simulink model "singlcontact_control_smc_lqr_mydimes_reaction"  (R2024a)
settings: Solver=VariableStepAuto  StartTime=0.0  StopTime=10  FixedStep=0.001  RelTol=1e-3
values from neighbouring files (symbols this model uses):
  ankle_servo_kd = 8    [robotParametersCtrl_mydiem_block_zmp.m]    (also in robotParametersCtrl_quad_modify_mydiem.m; robotParametersCtrl_quad_modify_mydiem_reaction.m)
  ankle_servo_ki = 4    [robotParametersCtrl_mydiem_block_zmp.m]    (also in robotParametersCtrl_quad_modify_mydiem.m; robotParametersCtrl_quad_modify_mydiem_reaction.m)
  ankle_servo_kp = 20    [robotParametersCtrl_mydiem_block_zmp.m]    (also in robotParametersCtrl_quad_modify_mydiem.m; robotParametersCtrl_quad_modify_mydiem_reaction.m)
  deriv_filter_coeff = 100    [robotParametersCtrl_mydiem_block_zmp.m]    (also in robotParametersCtrl_quad_modify_mydiem.m; robotParametersCtrl_quad_modify_mydiem_reaction.m)
  filter_coefficent_pid = 100    [robotParametersCtrl_mydiem_block_zmp.m]    (also in robotParametersCtrl_quad_modify_mydiem.m; robotParametersCtrl_quad_modify_mydiem_reaction.m)
  filter_coefficent_pids = 100    [robotParametersCtrl_quad_modify_mydiem_reaction.m]
  foot_z = 1.5    [robotParametersCtrl_mydiem_block_zmp.m]    (also in robotParametersCtrl_quad_modify_mydiem.m; robotParametersCtrl_quad_modify_mydiem_reaction.m)
  g = 9.81    [ABCDvalues_lqr_quad_mydime_reaction.m]    (also in robotParametersCtrl_mydiem_block_zmp.m = 9.80665; robotParametersCtrl_quad_modify_mydiem.m = 9.80665; robotParametersCtrl_quad_modify_mydiem_reaction.m = 9.80665)
  h = 32    [robotParametersCtrl_mydiem_block_zmp.m]    (also in robotParametersCtrl_quad_modify_mydiem.m; robotParametersCtrl_quad_modify_mydiem_reaction.m)
  height_plane = 0.025    [robotParametersCtrl_mydiem_block_zmp.m]    (also in robotParametersCtrl_quad_modify_mydiem.m; robotParametersCtrl_quad_modify_mydiem_reaction.m)
  hip_pitch_deriv = 20    [robotParametersCtrl_mydiem_block_zmp.m]    (also in robotParametersCtrl_quad_modify_mydiem.m = 200; robotParametersCtrl_quad_modify_mydiem_reaction.m = 200)
  hip_pitch_derivs = 200    [robotParametersCtrl_quad_modify_mydiem_reaction.m]
  hip_pitch_int = 0    [robotParametersCtrl_mydiem_block_zmp.m]    (also in robotParametersCtrl_quad_modify_mydiem.m = 150; robotParametersCtrl_quad_modify_mydiem_reaction.m = 150)
  hip_pitch_ints = 1500    [robotParametersCtrl_quad_modify_mydiem_reaction.m]
  hip_pitch_prop = 10    [robotParametersCtrl_mydiem_block_zmp.m]    (also in robotParametersCtrl_quad_modify_mydiem.m = 500; robotParametersCtrl_quad_modify_mydiem_reaction.m = 500)
  hip_pitch_props = 500    [robotParametersCtrl_quad_modify_mydiem_reaction.m]
  hip_roll_deriv = 28    [robotParametersCtrl_mydiem_block_zmp.m]    (also in robotParametersCtrl_quad_modify_mydiem.m = 280; robotParametersCtrl_quad_modify_mydiem_reaction.m = 280)
  hip_roll_derivs = 280    [robotParametersCtrl_quad_modify_mydiem_reaction.m]
  hip_roll_int = 0    [robotParametersCtrl_mydiem_block_zmp.m]    (also in robotParametersCtrl_quad_modify_mydiem.m = 180; robotParametersCtrl_quad_modify_mydiem_reaction.m = 180)
  hip_roll_ints = 180    [robotParametersCtrl_quad_modify_mydiem_reaction.m]
  hip_roll_prop = 10    [robotParametersCtrl_mydiem_block_zmp.m]    (also in robotParametersCtrl_quad_modify_mydiem.m = 300; robotParametersCtrl_quad_modify_mydiem_reaction.m = 300)
  hip_roll_props = 300    [robotParametersCtrl_quad_modify_mydiem_reaction.m]
  hip_servo_kd = 20    [robotParametersCtrl_mydiem_block_zmp.m]    (also in robotParametersCtrl_quad_modify_mydiem.m; robotParametersCtrl_quad_modify_mydiem_reaction.m)
  hip_servo_ki = 10    [robotParametersCtrl_mydiem_block_zmp.m]    (also in robotParametersCtrl_quad_modify_mydiem.m; robotParametersCtrl_quad_modify_mydiem_reaction.m)
  hip_servo_kp = 60    [robotParametersCtrl_mydiem_block_zmp.m]    (also in robotParametersCtrl_quad_modify_mydiem.m; robotParametersCtrl_quad_modify_mydiem_reaction.m)
  hip_smc_lamda = 85    [robotParametersCtrl_mydiem_block_zmp.m]    (also in robotParametersCtrl_quad_modify_mydiem.m; robotParametersCtrl_quad_modify_mydiem_reaction.m = 95)
  hip_smc_lamdas = 85    [robotParametersCtrl_quad_modify_mydiem_reaction.m]
  hip_smc_new = 25    [robotParametersCtrl_mydiem_block_zmp.m]    (also in robotParametersCtrl_quad_modify_mydiem.m; robotParametersCtrl_quad_modify_mydiem_reaction.m = 45)
  hip_smc_news = 25    [robotParametersCtrl_quad_modify_mydiem_reaction.m]
  init_angs_L = init_angs_R    [robotParametersCtrl_mydiem_block_zmp.m]    (also in robotParametersCtrl_quad_modify_mydiem.m; robotParametersCtrl_quad_modify_mydiem_reaction.m)
  init_angs_R = [0 -sum(init_angs) init_angs(2) 0 init_angs(1)]    [robotParametersCtrl_mydiem_block_zmp.m]    (also in robotParametersCtrl_quad_modify_mydiem.m; robotParametersCtrl_quad_modify_mydiem_reaction.m)
  init_height = h +                torso_z/2 + torso_offset_z + height_plane/2    (= 39.5125)    [robotParametersCtrl_mydiem_block_zmp.m]    (also in robotParametersCtrl_quad_modify_mydiem.m; robotParametersCtrl_quad_modify_mydiem_reaction.m)
  K = lqr(A, B, Q, R)    [ABCDvalues_lqr_quad_mydime_reaction.m]
  knee_pitch_deriv = 10    [robotParametersCtrl_mydiem_block_zmp.m]    (also in robotParametersCtrl_quad_modify_mydiem.m = 100; robotParametersCtrl_quad_modify_mydiem_reaction.m = 100)
  knee_pitch_derivs = 180    [robotParametersCtrl_quad_modify_mydiem_reaction.m]
  knee_pitch_int = 0    [robotParametersCtrl_mydiem_block_zmp.m]    (also in robotParametersCtrl_quad_modify_mydiem.m = 300; robotParametersCtrl_quad_modify_mydiem_reaction.m = 300)
  knee_pitch_ints = 7500    [robotParametersCtrl_quad_modify_mydiem_reaction.m]
  knee_pitch_prop = 10    [robotParametersCtrl_mydiem_block_zmp.m]    (also in robotParametersCtrl_quad_modify_mydiem.m = 400; robotParametersCtrl_quad_modify_mydiem_reaction.m = 400)
  knee_pitch_props = 1200    [robotParametersCtrl_quad_modify_mydiem_reaction.m]
  knee_servo_kd = 10    [robotParametersCtrl_mydiem_block_zmp.m]    (also in robotParametersCtrl_quad_modify_mydiem.m; robotParametersCtrl_quad_modify_mydiem_reaction.m)
  knee_servo_ki = 5    [robotParametersCtrl_mydiem_block_zmp.m]    (also in robotParametersCtrl_quad_modify_mydiem.m; robotParametersCtrl_quad_modify_mydiem_reaction.m)
  knee_servo_kp = 60    [robotParametersCtrl_mydiem_block_zmp.m]    (also in robotParametersCtrl_quad_modify_mydiem.m; robotParametersCtrl_quad_modify_mydiem_reaction.m)
  knee_smc_lamda = 140    [robotParametersCtrl_mydiem_block_zmp.m]    (also in robotParametersCtrl_quad_modify_mydiem.m; robotParametersCtrl_quad_modify_mydiem_reaction.m = 150)
  knee_smc_lamdas = 100    [robotParametersCtrl_quad_modify_mydiem_reaction.m]
  knee_smc_new = 80    [robotParametersCtrl_mydiem_block_zmp.m]    (also in robotParametersCtrl_quad_modify_mydiem.m; robotParametersCtrl_quad_modify_mydiem_reaction.m)
  knee_smc_news = 60    [robotParametersCtrl_quad_modify_mydiem_reaction.m]
  Kwalk = 0.6    [robotParametersCtrl_mydiem_block_zmp.m]    (also in robotParametersCtrl_quad_modify_mydiem.m; robotParametersCtrl_quad_modify_mydiem_reaction.m)
  l1 = 0.20    (= 0.2)    [ABCDvalues_lqr_quad_mydime_reaction.m]
  l2 = 0.20    (= 0.2)    [ABCDvalues_lqr_quad_mydime_reaction.m]
  lower_leg_length = 20    [robotParametersCtrl_mydiem_block_zmp.m]    (also in robotParametersCtrl_quad_modify_mydiem.m; robotParametersCtrl_quad_modify_mydiem_reaction.m)
  m1 = 0.45    [ABCDvalues_lqr_quad_mydime_reaction.m]
  m2 = 0.065    [ABCDvalues_lqr_quad_mydime_reaction.m]
  max_torque = 20    [robotParametersCtrl_mydiem_block_zmp.m]    (also in robotParametersCtrl_quad_modify_mydiem.m; robotParametersCtrl_quad_modify_mydiem_reaction.m)
  motion_time_constant = 0.01    [robotParametersCtrl_mydiem_block_zmp.m]    (also in robotParametersCtrl_quad_modify_mydiem.m; robotParametersCtrl_quad_modify_mydiem_reaction.m)
  plane_x = 25    [robotParametersCtrl_mydiem_block_zmp.m]    (also in robotParametersCtrl_quad_modify_mydiem.m; robotParametersCtrl_quad_modify_mydiem_reaction.m)
  plane_y = 3    [robotParametersCtrl_mydiem_block_zmp.m]    (also in robotParametersCtrl_quad_modify_mydiem.m; robotParametersCtrl_quad_modify_mydiem_reaction.m)
  stepHeight = 0.4    [ABCDvalues_lqr_quad_mydime_reaction.m]
  torso_offset_x = 17    [robotParametersCtrl_mydiem_block_zmp.m]    (also in robotParametersCtrl_quad_modify_mydiem.m; robotParametersCtrl_quad_modify_mydiem_reaction.m)
  torso_offset_x1 = -17    [robotParametersCtrl_mydiem_block_zmp.m]    (also in robotParametersCtrl_quad_modify_mydiem.m; robotParametersCtrl_quad_modify_mydiem_reaction.m)
  torso_offset_z = 0    [robotParametersCtrl_mydiem_block_zmp.m]    (also in robotParametersCtrl_quad_modify_mydiem.m; robotParametersCtrl_quad_modify_mydiem_reaction.m)
  torso_x = 40    [robotParametersCtrl_mydiem_block_zmp.m]    (also in robotParametersCtrl_quad_modify_mydiem.m; robotParametersCtrl_quad_modify_mydiem_reaction.m)
  torso_y = 20    [robotParametersCtrl_mydiem_block_zmp.m]    (also in robotParametersCtrl_quad_modify_mydiem.m; robotParametersCtrl_quad_modify_mydiem_reaction.m)
  torso_z = 15    [robotParametersCtrl_mydiem_block_zmp.m]    (also in robotParametersCtrl_quad_modify_mydiem.m; robotParametersCtrl_quad_modify_mydiem_reaction.m)
  Ts = 0.05    [ABCDvalues_lqr_quad_mydime_reaction.m]
  TsCtrl = 0.05    [robotParametersCtrl_mydiem_block_zmp.m]    (also in robotParametersCtrl_quad_modify_mydiem.m; robotParametersCtrl_quad_modify_mydiem_reaction.m)
  tWalk = 0.3    [robotParametersCtrl_mydiem_block_zmp.m]    (also in robotParametersCtrl_quad_modify_mydiem.m; robotParametersCtrl_quad_modify_mydiem_reaction.m)
  upper_leg_length = 20    [robotParametersCtrl_mydiem_block_zmp.m]    (also in robotParametersCtrl_quad_modify_mydiem.m; robotParametersCtrl_quad_modify_mydiem_reaction.m)
undefined symbols (not defined in the file or in its folder): X, Y, Z
libraries: simulink_extras x256, slpidlib x128, sm_lib x71, simulink x43, nesl_utility x35, walkingRobotUtils x21, dspsrcs4 x18, dspobslib x8
(part 31 of 33)

== system singlcontact_control_smc_lqr_mydimes_reaction/Walking Robot/smc+neuro+distur1/SMC Controllers FR2/Equivalent control/SMC equivalent T1 ==
  theta2 : Inport
  theta1 : Inport  Port=2
  theta2ddot : Inport  Port=3
  theta1dot : Inport  Port=4
  theta2dot : Inport  Port=5
  theta1ddot : Inport  Port=6
  Add{1..4} (4 alike) : Sum
  Add5 : Sum  Inputs=+--+++
  Add6 : Sum  Inputs=++++
  Constant : Constant  Value=0.3
  Constant10 : Constant  Value=m2*l1^2
  Constant11 : Constant  Value=0.3*m1*l1^2
  Constant12 : Constant  Value=m2*l1*l2
  Constant2 : Constant  Value=0.5
  Constant3 : Constant
  Constant4 : Constant  Value=0.5
  Constant5 : Constant
  Constant6 : Constant  Value=g*l1
  Constant7 : Constant  Value=0.5
  Constant9 : Constant  Value=0.3*m2*l2^2
  Cos : Trigonometry  Operator=cos
  Cos1 : Trigonometry  Operator=cos
  Gain1 : Gain  Gain=m2*l2^2
  Gain2 : Gain  Gain=m2*l2*l1
  Gain4 : Gain  Gain=m2*l2*l1
  Gain6 : Gain  Gain=m1
  Gain7 : Gain  Gain=m2
  Gain8 : Gain  Gain=m2*g*l2
  Product{1..3,7..9} (6 alike) : Product
  Product4 : Product  Inputs=4
  Product5 : Product  Inputs=3
  Product6 : Product  Inputs=3
  Sin : Trigonometry
  Sin1 : Trigonometry
  Sin2 : Trigonometry
  Square1 : Math  Operator=square
  T1 : Outport
  wires:
  Add2/1 -> Product1/1
  Product9/1 -> Add2/2
  [lamdaBR1] -> Product9/1
  [edotBR1] -> Product9/2
  Add5/1 -> T1/1
  Product1/1 -> Add5/6
  theta1ddot/1 -> Add2/1
  Add6/1 -> Product1/2
  Product8/1 -> Add6/1
  Constant11/1 -> Add6/2
  Constant10/1 -> Add6/4
  Constant9/1 -> Add6/3
  Cos1/1 -> Product8/1
  Constant12/1 -> Product8/2  "X_dd"
  theta2/1 -> Cos/1, Sin/1, Add4/1, Cos1/1
  Product7/1 -> Add5/5
  Product6/1 -> Add5/4
  Product5/1 -> Add5/3
  Product4/1 -> Add5/2
  Product3/1 -> Add5/1
  Sin2/1 -> Product7/2
  Gain8/1 -> Product7/1
  Add4/1 -> Sin2/1
  Constant7/1 -> Gain8/1
  Constant6/1 -> Product6/3
  Sin1/1 -> Product6/2
  Add3/1 -> Product6/1
  theta1/1 -> Sin1/1, Add4/2
  Gain6/1 -> Add3/1
  Gain7/1 -> Add3/2
  Constant5/1 -> Gain7/1
  Constant4/1 -> Gain6/1
  Square1/1 -> Product5/3
  Constant3/1 -> Gain4/1
  Gain4/1 -> Product4/1
  Sin/1 -> Product5/2, Product4/2
  theta2dot/1 -> Square1/1, Product4/4
  theta1dot/1 -> Product4/3
  Add1/1 -> Product3/2
  theta2ddot/1 -> Product3/1
  Product2/1 -> Add1/2
  Gain1/1 -> Add1/1
  Gain2/1 -> Product5/1, Product2/1
  Cos/1 -> Product2/2
  Constant2/1 -> Gain2/1
  Constant/1 -> Gain1/1

== system singlcontact_control_smc_lqr_mydimes_reaction/Walking Robot/smc+neuro+distur1/SMC Controllers FR2/Equivalent control/SMC equivalent T2 ==
  theta1ddot : Inport
  theta2 : Inport  Port=2
  theta1 : Inport  Port=3
  theta2ddot : Inport  Port=4
  theta1dot : Inport  Port=5
  Add1 : Sum
  Add2 : Sum
  Add4 : Sum
  Add5 : Sum  Inputs=++++
  Constant : Constant  Value=0.5
  Constant1 : Constant  Value=0.3
  Constant2 : Constant  Value=0.5
  Constant3 : Constant
  Gain10 : Gain  Gain=m2*l2^2
  Gain11 : Gain  Gain=m2*l2
  Gain12 : Gain  Gain=g
  Gain13 : Gain  Gain=(1/3)*(m2*(l2^2))
  Gain5 : Gain  Gain=m2*l1*l2
  Product{1..4,7} (5 alike) : Product
  Product6 : Product  Inputs=3
  Sin : Trigonometry
  Square3 : Math  Operator=square
  Trigonometric Function3 : Trigonometry  Operator=cos
  Trigonometric Function4 : Trigonometry
  T2 : Outport
  wires:
  Product2/1 -> Add5/4
  Gain13/1 -> Product2/1
  Add1/1 -> Product2/2
  Constant3/1 -> Gain13/1
  theta2ddot/1 -> Add1/2
  [edotBR2] -> Product1/1
  [lamdaBR2] -> Product1/2
  Product1/1 -> Add1/1
  Add5/1 -> T2/1
  Product7/1 -> Add5/3
  Product6/1 -> Add5/2
  Product4/1 -> Add5/1
  Add4/1 -> Sin/1
  Sin/1 -> Product7/2
  theta1/1 -> Add4/1
  Gain12/1 -> Product7/1
  Gain11/1 -> Gain12/1
  Constant2/1 -> Gain11/1
  Square3/1 -> Product6/3
  theta1dot/1 -> Square3/1
  Trigonometric Function4/1 -> Product6/2
  Constant1/1 -> Gain10/1
  Constant/1 -> Gain5/1
  theta1ddot/1 -> Product4/1
  Add2/1 -> Product4/2
  Gain10/1 -> Add2/2
  Product3/1 -> Add2/1
  Gain5/1 -> Product6/1, Product3/2
  Trigonometric Function3/1 -> Product3/1
  theta2/1 -> Trigonometric Function4/1, Add4/2, Trigonometric Function3/1

== system singlcontact_control_smc_lqr_mydimes_reaction/Walking Robot/smc+neuro+distur1/SMC Controllers FR3/Equivalent control/SMC equivalent T1 ==
  theta2 : Inport
  theta1 : Inport  Port=2
  theta2ddot : Inport  Port=3
  theta1dot : Inport  Port=4
  theta2dot : Inport  Port=5
  theta1ddot : Inport  Port=6
  Add{1..4} (4 alike) : Sum
  Add5 : Sum  Inputs=+--+++
  Add6 : Sum  Inputs=++++
  Constant : Constant  Value=0.3
  Constant10 : Constant  Value=m2*l1^2
  Constant11 : Constant  Value=0.3*m1*l1^2
  Constant12 : Constant  Value=m2*l1*l2
  Constant2 : Constant  Value=0.5
  Constant3 : Constant
  Constant4 : Constant  Value=0.5
  Constant5 : Constant
  Constant6 : Constant  Value=g*l1
  Constant7 : Constant  Value=0.5
  Constant9 : Constant  Value=0.3*m2*l2^2
  Cos : Trigonometry  Operator=cos
  Cos1 : Trigonometry  Operator=cos
  Gain1 : Gain  Gain=m2*l2^2
  Gain2 : Gain  Gain=m2*l2*l1
  Gain4 : Gain  Gain=m2*l2*l1
  Gain6 : Gain  Gain=m1
  Gain7 : Gain  Gain=m2
  Gain8 : Gain  Gain=m2*g*l2
  Product{1..3,7..9} (6 alike) : Product
  Product4 : Product  Inputs=4
  Product5 : Product  Inputs=3
  Product6 : Product  Inputs=3
  Sin : Trigonometry
  Sin1 : Trigonometry
  Sin2 : Trigonometry
  Square1 : Math  Operator=square
  T1 : Outport
  wires:
  Constant/1 -> Gain1/1
  Constant2/1 -> Gain2/1
  Cos/1 -> Product2/2
  Gain2/1 -> Product2/1, Product5/1
  Gain1/1 -> Add1/1
  Product2/1 -> Add1/2
  theta2ddot/1 -> Product3/1
  Add1/1 -> Product3/2
  theta1dot/1 -> Product4/3
  theta2dot/1 -> Product4/4, Square1/1
  Sin/1 -> Product4/2, Product5/2
  Gain4/1 -> Product4/1
  Constant3/1 -> Gain4/1
  Square1/1 -> Product5/3
  Constant4/1 -> Gain6/1
  Constant5/1 -> Gain7/1
  Gain7/1 -> Add3/2
  Gain6/1 -> Add3/1
  theta1/1 -> Add4/2, Sin1/1
  Add3/1 -> Product6/1
  Sin1/1 -> Product6/2
  Constant6/1 -> Product6/3
  Constant7/1 -> Gain8/1
  Add4/1 -> Sin2/1
  Gain8/1 -> Product7/1
  Sin2/1 -> Product7/2
  Product3/1 -> Add5/1
  Product4/1 -> Add5/2
  Product5/1 -> Add5/3
  Product6/1 -> Add5/4
  Product7/1 -> Add5/5
  theta2/1 -> Cos1/1, Add4/1, Sin/1, Cos/1
  Constant12/1 -> Product8/2  "X_dd"
  Cos1/1 -> Product8/1
  Constant9/1 -> Add6/3
  Constant10/1 -> Add6/4
  Constant11/1 -> Add6/2
  Product8/1 -> Add6/1
  Add6/1 -> Product1/2
  theta1ddot/1 -> Add2/1
  Product1/1 -> Add5/6
  Add5/1 -> T1/1
  [edotBL1] -> Product9/2
  [lamdaBL1] -> Product9/1
  Product9/1 -> Add2/2
  Add2/1 -> Product1/1

== system singlcontact_control_smc_lqr_mydimes_reaction/Walking Robot/smc+neuro+distur1/SMC Controllers FR3/Equivalent control/SMC equivalent T2 ==
  theta1ddot : Inport
  theta2 : Inport  Port=2
  theta1 : Inport  Port=3
  theta2ddot : Inport  Port=4
  theta1dot : Inport  Port=5
  Add1 : Sum
  Add2 : Sum
  Add4 : Sum
  Add5 : Sum  Inputs=++++
  Constant : Constant  Value=0.5
  Constant1 : Constant  Value=0.3
  Constant2 : Constant  Value=0.5
  Constant3 : Constant
  Gain10 : Gain  Gain=m2*l2^2
  Gain11 : Gain  Gain=m2*l2
  Gain12 : Gain  Gain=g
  Gain13 : Gain  Gain=(1/3)*(m2*(l2^2))
  Gain5 : Gain  Gain=m2*l1*l2
  Product{1..4,7} (5 alike) : Product
  Product6 : Product  Inputs=3
  Sin : Trigonometry
  Square3 : Math  Operator=square
  Trigonometric Function3 : Trigonometry  Operator=cos
  Trigonometric Function4 : Trigonometry
  T2 : Outport
  wires:
  theta2/1 -> Trigonometric Function3/1, Add4/2, Trigonometric Function4/1
  Trigonometric Function3/1 -> Product3/1
  Gain5/1 -> Product3/2, Product6/1
  Product3/1 -> Add2/1
  Gain10/1 -> Add2/2
  Add2/1 -> Product4/2
  theta1ddot/1 -> Product4/1
  Constant/1 -> Gain5/1
  Constant1/1 -> Gain10/1
  Trigonometric Function4/1 -> Product6/2
  theta1dot/1 -> Square3/1
  Square3/1 -> Product6/3
  Constant2/1 -> Gain11/1
  Gain11/1 -> Gain12/1
  Gain12/1 -> Product7/1
  theta1/1 -> Add4/1
  Sin/1 -> Product7/2
  Add4/1 -> Sin/1
  Product4/1 -> Add5/1
  Product6/1 -> Add5/2
  Product7/1 -> Add5/3
  Add5/1 -> T2/1
  Product1/1 -> Add1/1
  [lamdaBL2] -> Product1/2
  [edotBL2] -> Product1/1
  theta2ddot/1 -> Add1/2
  Constant3/1 -> Gain13/1
  Add1/1 -> Product2/2
  Gain13/1 -> Product2/1
  Product2/1 -> Add5/4

== system singlcontact_control_smc_lqr_mydimes_reaction/Walking Robot/smc+neuro1+reaction/SMC Controllers BL/Equivalent control/SMC equivalent T1 ==
  theta2 : Inport
  theta1 : Inport  Port=2
  theta2ddot : Inport  Port=3
  theta1dot : Inport  Port=4
  theta2dot : Inport  Port=5
  theta1ddot : Inport  Port=6
  Add{1..4} (4 alike) : Sum
  Add5 : Sum  Inputs=+--+++
  Add6 : Sum  Inputs=++++
  Constant : Constant  Value=0.3
  Constant10 : Constant  Value=m2*l1^2
  Constant11 : Constant  Value=0.3*m1*l1^2
  Constant12 : Constant  Value=m2*l1*l2
  Constant2 : Constant  Value=0.5
  Constant3 : Constant
  Constant4 : Constant  Value=0.5
  Constant5 : Constant
  Constant6 : Constant  Value=g*l1
  Constant7 : Constant  Value=0.5
  Constant9 : Constant  Value=0.3*m2*l2^2
  Cos : Trigonometry  Operator=cos
  Cos1 : Trigonometry  Operator=cos
  Gain1 : Gain  Gain=m2*l2^2
  Gain2 : Gain  Gain=m2*l2*l1
  Gain4 : Gain  Gain=m2*l2*l1
  Gain6 : Gain  Gain=m1
  Gain7 : Gain  Gain=m2
  Gain8 : Gain  Gain=m2*g*l2
  Product{1..3,7..9} (6 alike) : Product
  Product4 : Product  Inputs=4
  Product5 : Product  Inputs=3
  Product6 : Product  Inputs=3
  Sin : Trigonometry
  Sin1 : Trigonometry
  Sin2 : Trigonometry
  Square1 : Math  Operator=square
  T1 : Outport
  wires:
  Add2/1 -> Product1/1
  Product9/1 -> Add2/2
  [lamdaBL1] -> Product9/1
  [edotBL1] -> Product9/2
  Add5/1 -> T1/1
  Product1/1 -> Add5/6
  theta1ddot/1 -> Add2/1
  Add6/1 -> Product1/2
  Product8/1 -> Add6/1
  Constant11/1 -> Add6/2
  Constant10/1 -> Add6/4
  Constant9/1 -> Add6/3
  Cos1/1 -> Product8/1
  Constant12/1 -> Product8/2  "X_dd"
  theta2/1 -> Cos/1, Sin/1, Add4/1, Cos1/1
  Product7/1 -> Add5/5
  Product6/1 -> Add5/4
  Product5/1 -> Add5/3
  Product4/1 -> Add5/2
  Product3/1 -> Add5/1
  Sin2/1 -> Product7/2
  Gain8/1 -> Product7/1
  Add4/1 -> Sin2/1
  Constant7/1 -> Gain8/1
  Constant6/1 -> Product6/3
  Sin1/1 -> Product6/2
  Add3/1 -> Product6/1
  theta1/1 -> Sin1/1, Add4/2
  Gain6/1 -> Add3/1
  Gain7/1 -> Add3/2
  Constant5/1 -> Gain7/1
  Constant4/1 -> Gain6/1
  Square1/1 -> Product5/3
  Constant3/1 -> Gain4/1
  Gain4/1 -> Product4/1
  Sin/1 -> Product5/2, Product4/2
  theta2dot/1 -> Square1/1, Product4/4
  theta1dot/1 -> Product4/3
  Add1/1 -> Product3/2
  theta2ddot/1 -> Product3/1
  Product2/1 -> Add1/2
  Gain1/1 -> Add1/1
  Gain2/1 -> Product5/1, Product2/1
  Cos/1 -> Product2/2
  Constant2/1 -> Gain2/1
  Constant/1 -> Gain1/1

== system singlcontact_control_smc_lqr_mydimes_reaction/Walking Robot/smc+neuro1+reaction/SMC Controllers BL/Equivalent control/SMC equivalent T2 ==
  theta1ddot : Inport
  theta2 : Inport  Port=2
  theta1 : Inport  Port=3
  theta2ddot : Inport  Port=4
  theta1dot : Inport  Port=5
  Add1 : Sum
  Add2 : Sum
  Add4 : Sum
  Add5 : Sum  Inputs=++++
  Constant : Constant  Value=0.5
  Constant1 : Constant  Value=0.3
  Constant2 : Constant  Value=0.5
  Constant3 : Constant
  Gain10 : Gain  Gain=m2*l2^2
  Gain11 : Gain  Gain=m2*l2
  Gain12 : Gain  Gain=g
  Gain13 : Gain  Gain=(1/3)*(m2*(l2^2))
  Gain5 : Gain  Gain=m2*l1*l2
  Product{1..4,7} (5 alike) : Product
  Product6 : Product  Inputs=3
  Sin : Trigonometry
  Square3 : Math  Operator=square
  Trigonometric Function3 : Trigonometry  Operator=cos
  Trigonometric Function4 : Trigonometry
  T2 : Outport
  wires:
  Product2/1 -> Add5/4
  Gain13/1 -> Product2/1
  Add1/1 -> Product2/2
  Constant3/1 -> Gain13/1
  theta2ddot/1 -> Add1/2
  [edotBL2] -> Product1/1
  [lamdaBL2] -> Product1/2
  Product1/1 -> Add1/1
  Add5/1 -> T2/1
  Product7/1 -> Add5/3
  Product6/1 -> Add5/2
  Product4/1 -> Add5/1
  Add4/1 -> Sin/1
  Sin/1 -> Product7/2
  theta1/1 -> Add4/1
  Gain12/1 -> Product7/1
  Gain11/1 -> Gain12/1
  Constant2/1 -> Gain11/1
  Square3/1 -> Product6/3
  theta1dot/1 -> Square3/1
  Trigonometric Function4/1 -> Product6/2
  Constant1/1 -> Gain10/1
  Constant/1 -> Gain5/1
  theta1ddot/1 -> Product4/1
  Add2/1 -> Product4/2
  Gain10/1 -> Add2/2
  Product3/1 -> Add2/1
  Gain5/1 -> Product6/1, Product3/2
  Trigonometric Function3/1 -> Product3/1
  theta2/1 -> Trigonometric Function4/1, Add4/2, Trigonometric Function3/1

== system singlcontact_control_smc_lqr_mydimes_reaction/Walking Robot/smc+neuro1+reaction/SMC Controllers BL/Subsystem2/length from ground ==
  In1 : Inport
  In2 : Inport  Port=2
  Gain1 : Gain  Gain=l1
  Gain3 : Gain  Gain=l1
  Gain4 : Gain  Gain=l2
  Sin : Trigonometry
  Sin1 : Trigonometry
  Sin3 : Trigonometry
  Sum : Sum  Inputs=|++
  Sum2 : Sum  Inputs=|++
  Output : Outport
  Outport : Outport  Port=2
  wires:
  In1/1 -> Sin/1, Sum2/1, Sin1/1
  Sin/1 -> Gain1/1
  Sum/1 -> Outport/1
  Gain4/1 -> Sum/2
  Gain3/1 -> Sum/1
  Sum2/1 -> Sin3/1
  Sin1/1 -> Gain3/1
  Gain1/1 -> Output/1
  Sin3/1 -> Gain4/1
  In2/1 -> Sum2/2

== system singlcontact_control_smc_lqr_mydimes_reaction/Walking Robot/smc+neuro1+reaction/SMC Controllers BR/Equivalent control/SMC equivalent T1 ==
  theta2 : Inport
  theta1 : Inport  Port=2
  theta2ddot : Inport  Port=3
  theta1dot : Inport  Port=4
  theta2dot : Inport  Port=5
  theta1ddot : Inport  Port=6
  Add{1..4} (4 alike) : Sum
  Add5 : Sum  Inputs=+--+++
  Add6 : Sum  Inputs=++++
  Constant : Constant  Value=0.3
  Constant10 : Constant  Value=m2*l1^2
  Constant11 : Constant  Value=0.3*m1*l1^2
  Constant12 : Constant  Value=m2*l1*l2
  Constant2 : Constant  Value=0.5
  Constant3 : Constant
  Constant4 : Constant  Value=0.5
  Constant5 : Constant
  Constant6 : Constant  Value=g*l1
  Constant7 : Constant  Value=0.5
  Constant9 : Constant  Value=0.3*m2*l2^2
  Cos : Trigonometry  Operator=cos
  Cos1 : Trigonometry  Operator=cos
  Gain1 : Gain  Gain=m2*l2^2
  Gain2 : Gain  Gain=m2*l2*l1
  Gain4 : Gain  Gain=m2*l2*l1
  Gain6 : Gain  Gain=m1
  Gain7 : Gain  Gain=m2
  Gain8 : Gain  Gain=m2*g*l2
  Product{1..3,7..9} (6 alike) : Product
  Product4 : Product  Inputs=4
  Product5 : Product  Inputs=3
  Product6 : Product  Inputs=3
  Sin : Trigonometry
  Sin1 : Trigonometry
  Sin2 : Trigonometry
  Square1 : Math  Operator=square
  T1 : Outport
  wires:
  Constant/1 -> Gain1/1
  Constant2/1 -> Gain2/1
  Cos/1 -> Product2/2
  Gain2/1 -> Product2/1, Product5/1
  Gain1/1 -> Add1/1
  Product2/1 -> Add1/2
  theta2ddot/1 -> Product3/1
  Add1/1 -> Product3/2
  theta1dot/1 -> Product4/3
  theta2dot/1 -> Product4/4, Square1/1
  Sin/1 -> Product4/2, Product5/2
  Gain4/1 -> Product4/1
  Constant3/1 -> Gain4/1
  Square1/1 -> Product5/3
  Constant4/1 -> Gain6/1
  Constant5/1 -> Gain7/1
  Gain7/1 -> Add3/2
  Gain6/1 -> Add3/1
  theta1/1 -> Add4/2, Sin1/1
  Add3/1 -> Product6/1
  Sin1/1 -> Product6/2
  Constant6/1 -> Product6/3
  Constant7/1 -> Gain8/1
  Add4/1 -> Sin2/1
  Gain8/1 -> Product7/1
  Sin2/1 -> Product7/2
  Product3/1 -> Add5/1
  Product4/1 -> Add5/2
  Product5/1 -> Add5/3
  Product6/1 -> Add5/4
  Product7/1 -> Add5/5
  theta2/1 -> Cos1/1, Add4/1, Sin/1, Cos/1
  Constant12/1 -> Product8/2  "X_dd"
  Cos1/1 -> Product8/1
  Constant9/1 -> Add6/3
  Constant10/1 -> Add6/4
  Constant11/1 -> Add6/2
  Product8/1 -> Add6/1
  Add6/1 -> Product1/2
  theta1ddot/1 -> Add2/1
  Product1/1 -> Add5/6
  Add5/1 -> T1/1
  [edotBR1] -> Product9/2
  [lamdaBR1] -> Product9/1
  Product9/1 -> Add2/2
  Add2/1 -> Product1/1

== system singlcontact_control_smc_lqr_mydimes_reaction/Walking Robot/smc+neuro1+reaction/SMC Controllers BR/Equivalent control/SMC equivalent T2 ==
  theta1ddot : Inport
  theta2 : Inport  Port=2
  theta1 : Inport  Port=3
  theta2ddot : Inport  Port=4
  theta1dot : Inport  Port=5
  Add1 : Sum
  Add2 : Sum
  Add4 : Sum
  Add5 : Sum  Inputs=++++
  Constant : Constant  Value=0.5
  Constant1 : Constant  Value=0.3
  Constant2 : Constant  Value=0.5
  Constant3 : Constant
  Gain10 : Gain  Gain=m2*l2^2
  Gain11 : Gain  Gain=m2*l2
  Gain12 : Gain  Gain=g
  Gain13 : Gain  Gain=(1/3)*(m2*(l2^2))
  Gain5 : Gain  Gain=m2*l1*l2
  Product{1..4,7} (5 alike) : Product
  Product6 : Product  Inputs=3
  Sin : Trigonometry
  Square3 : Math  Operator=square
  Trigonometric Function3 : Trigonometry  Operator=cos
  Trigonometric Function4 : Trigonometry
  T2 : Outport
  wires:
  theta2/1 -> Trigonometric Function3/1, Add4/2, Trigonometric Function4/1
  Trigonometric Function3/1 -> Product3/1
  Gain5/1 -> Product3/2, Product6/1
  Product3/1 -> Add2/1
  Gain10/1 -> Add2/2
  Add2/1 -> Product4/2
  theta1ddot/1 -> Product4/1
  Constant/1 -> Gain5/1
  Constant1/1 -> Gain10/1
  Trigonometric Function4/1 -> Product6/2
  theta1dot/1 -> Square3/1
  Square3/1 -> Product6/3
  Constant2/1 -> Gain11/1
  Gain11/1 -> Gain12/1
  Gain12/1 -> Product7/1
  theta1/1 -> Add4/1
  Sin/1 -> Product7/2
  Add4/1 -> Sin/1
  Product4/1 -> Add5/1
  Product6/1 -> Add5/2
  Product7/1 -> Add5/3
  Add5/1 -> T2/1
  Product1/1 -> Add1/1
  [lamdaBR2] -> Product1/2
  [edotBR2] -> Product1/1
  theta2ddot/1 -> Add1/2
  Constant3/1 -> Gain13/1
  Add1/1 -> Product2/2
  Gain13/1 -> Product2/1
  Product2/1 -> Add5/4

== system singlcontact_control_smc_lqr_mydimes_reaction/Walking Robot/smc+neuro1+reaction/SMC Controllers BR/Subsystem2/length from ground ==
  In1 : Inport
  In2 : Inport  Port=2
  Gain1 : Gain  Gain=l1
  Gain3 : Gain  Gain=l1
  Gain4 : Gain  Gain=l2
  Sin : Trigonometry
  Sin1 : Trigonometry
  Sin3 : Trigonometry
  Sum : Sum  Inputs=|++
  Sum2 : Sum  Inputs=|++
  Output : Outport
  Outport : Outport  Port=2
  wires:
  In1/1 -> Sin/1, Sum2/1, Sin1/1
  Sin/1 -> Gain1/1
  Sum/1 -> Outport/1
  Gain4/1 -> Sum/2
  Gain3/1 -> Sum/1
  Sum2/1 -> Sin3/1
  Sin1/1 -> Gain3/1
  Gain1/1 -> Output/1
  Sin3/1 -> Gain4/1
  In2/1 -> Sum2/2

== system singlcontact_control_smc_lqr_mydimes_reaction/Walking Robot/smc+neuro1+reaction/SMC Controllers FL/Equivalent control/SMC equivalent T1 ==
  theta2 : Inport
  theta1 : Inport  Port=2
  theta2ddot : Inport  Port=3
  theta1dot : Inport  Port=4
  theta2dot : Inport  Port=5
  theta1ddot : Inport  Port=6
  Add{1..4} (4 alike) : Sum
  Add5 : Sum  Inputs=+--+++
  Add6 : Sum  Inputs=++++
  Constant : Constant  Value=0.3
  Constant10 : Constant  Value=m2*l1^2
  Constant11 : Constant  Value=0.3*m1*l1^2
  Constant12 : Constant  Value=m2*l1*l2
  Constant2 : Constant  Value=0.5
  Constant3 : Constant
  Constant4 : Constant  Value=0.5
  Constant5 : Constant
  Constant6 : Constant  Value=g*l1
  Constant7 : Constant  Value=0.5
  Constant9 : Constant  Value=0.3*m2*l2^2
  Cos : Trigonometry  Operator=cos
  Cos1 : Trigonometry  Operator=cos
  Gain1 : Gain  Gain=m2*l2^2
  Gain2 : Gain  Gain=m2*l2*l1
  Gain4 : Gain  Gain=m2*l2*l1
  Gain6 : Gain  Gain=m1
  Gain7 : Gain  Gain=m2
  Gain8 : Gain  Gain=m2*g*l2
  Product{1..3,7..9} (6 alike) : Product
  Product4 : Product  Inputs=4
  Product5 : Product  Inputs=3
  Product6 : Product  Inputs=3
  Sin : Trigonometry
  Sin1 : Trigonometry
  Sin2 : Trigonometry
  Square1 : Math  Operator=square
  T1 : Outport
  wires:
  Add2/1 -> Product1/1
  Product9/1 -> Add2/2
  [lamdaFL1] -> Product9/1
  [edotFL1] -> Product9/2
  Add5/1 -> T1/1
  Product1/1 -> Add5/6
  theta1ddot/1 -> Add2/1
  Add6/1 -> Product1/2
  Product8/1 -> Add6/1
  Constant11/1 -> Add6/2
  Constant10/1 -> Add6/4
  Constant9/1 -> Add6/3
  Cos1/1 -> Product8/1
  Constant12/1 -> Product8/2  "X_dd"
  theta2/1 -> Cos/1, Sin/1, Add4/1, Cos1/1
  Product7/1 -> Add5/5
  Product6/1 -> Add5/4
  Product5/1 -> Add5/3
  Product4/1 -> Add5/2
  Product3/1 -> Add5/1
  Sin2/1 -> Product7/2
  Gain8/1 -> Product7/1
  Add4/1 -> Sin2/1
  Constant7/1 -> Gain8/1
  Constant6/1 -> Product6/3
  Sin1/1 -> Product6/2
  Add3/1 -> Product6/1
  theta1/1 -> Sin1/1, Add4/2
  Gain6/1 -> Add3/1
  Gain7/1 -> Add3/2
  Constant5/1 -> Gain7/1
  Constant4/1 -> Gain6/1
  Square1/1 -> Product5/3
  Constant3/1 -> Gain4/1
  Gain4/1 -> Product4/1
  Sin/1 -> Product5/2, Product4/2
  theta2dot/1 -> Square1/1, Product4/4
  theta1dot/1 -> Product4/3
  Add1/1 -> Product3/2
  theta2ddot/1 -> Product3/1
  Product2/1 -> Add1/2
  Gain1/1 -> Add1/1
  Gain2/1 -> Product5/1, Product2/1
  Cos/1 -> Product2/2
  Constant2/1 -> Gain2/1
  Constant/1 -> Gain1/1

== system singlcontact_control_smc_lqr_mydimes_reaction/Walking Robot/smc+neuro1+reaction/SMC Controllers FL/Equivalent control/SMC equivalent T2 ==
  theta1ddot : Inport
  theta2 : Inport  Port=2
  theta1 : Inport  Port=3
  theta2ddot : Inport  Port=4
  theta1dot : Inport  Port=5
  Add1 : Sum
  Add2 : Sum
  Add4 : Sum
  Add5 : Sum  Inputs=++++
  Constant : Constant  Value=0.5
  Constant1 : Constant  Value=0.3
  Constant2 : Constant  Value=0.5
  Constant3 : Constant
  Gain10 : Gain  Gain=m2*l2^2
  Gain11 : Gain  Gain=m2*l2
  Gain12 : Gain  Gain=g
  Gain13 : Gain  Gain=(1/3)*(m2*(l2^2))
  Gain5 : Gain  Gain=m2*l1*l2
  Product{1..4,7} (5 alike) : Product
  Product6 : Product  Inputs=3
  Sin : Trigonometry
  Square3 : Math  Operator=square
  Trigonometric Function3 : Trigonometry  Operator=cos
  Trigonometric Function4 : Trigonometry
  T2 : Outport
  wires:
  Product2/1 -> Add5/4
  Gain13/1 -> Product2/1
  Add1/1 -> Product2/2
  Constant3/1 -> Gain13/1
  theta2ddot/1 -> Add1/2
  [edotFL2] -> Product1/1
  [lamdaFL2] -> Product1/2
  Product1/1 -> Add1/1
  Add5/1 -> T2/1
  Product7/1 -> Add5/3
  Product6/1 -> Add5/2
  Product4/1 -> Add5/1
  Add4/1 -> Sin/1
  Sin/1 -> Product7/2
  theta1/1 -> Add4/1
  Gain12/1 -> Product7/1
  Gain11/1 -> Gain12/1
  Constant2/1 -> Gain11/1
  Square3/1 -> Product6/3
  theta1dot/1 -> Square3/1
  Trigonometric Function4/1 -> Product6/2
  Constant1/1 -> Gain10/1
  Constant/1 -> Gain5/1
  theta1ddot/1 -> Product4/1
  Add2/1 -> Product4/2
  Gain10/1 -> Add2/2
  Product3/1 -> Add2/1
  Gain5/1 -> Product6/1, Product3/2
  Trigonometric Function3/1 -> Product3/1
  theta2/1 -> Trigonometric Function4/1, Add4/2, Trigonometric Function3/1

== system singlcontact_control_smc_lqr_mydimes_reaction/Walking Robot/smc+neuro1+reaction/SMC Controllers FL/Subsystem2/length from ground ==
  In1 : Inport
  In2 : Inport  Port=2
  Gain1 : Gain  Gain=l1
  Gain3 : Gain  Gain=l1
  Gain4 : Gain  Gain=l2
  Sin : Trigonometry
  Sin1 : Trigonometry
  Sin3 : Trigonometry
  Sum : Sum  Inputs=|++
  Sum2 : Sum  Inputs=|++
  Output : Outport
  Outport : Outport  Port=2
  wires:
  In1/1 -> Sin/1, Sum2/1, Sin1/1
  Sin/1 -> Gain1/1
  Sum/1 -> Outport/1
  Gain4/1 -> Sum/2
  Gain3/1 -> Sum/1
  Sum2/1 -> Sin3/1
  Sin1/1 -> Gain3/1
  Gain1/1 -> Output/1
  Sin3/1 -> Gain4/1
  In2/1 -> Sum2/2

== system singlcontact_control_smc_lqr_mydimes_reaction/Walking Robot/smc+neuro1+reaction/SMC Controllers FR/Equivalent control/SMC equivalent T1 ==
  theta2 : Inport
  theta1 : Inport  Port=2
  theta2ddot : Inport  Port=3
  theta1dot : Inport  Port=4
  theta2dot : Inport  Port=5
  theta1ddot : Inport  Port=6
  Add{1..4} (4 alike) : Sum
  Add5 : Sum  Inputs=+--+++
  Add6 : Sum  Inputs=++++
  Constant : Constant  Value=0.3
  Constant10 : Constant  Value=m2*l1^2
  Constant11 : Constant  Value=0.3*m1*l1^2
  Constant12 : Constant  Value=m2*l1*l2
  Constant2 : Constant  Value=0.5
  Constant3 : Constant
  Constant4 : Constant  Value=0.5
  Constant5 : Constant
  Constant6 : Constant  Value=g*l1
  Constant7 : Constant  Value=0.5
  Constant9 : Constant  Value=0.3*m2*l2^2
  Cos : Trigonometry  Operator=cos
  Cos1 : Trigonometry  Operator=cos
  Gain1 : Gain  Gain=m2*l2^2
  Gain2 : Gain  Gain=m2*l2*l1
  Gain4 : Gain  Gain=m2*l2*l1
  Gain6 : Gain  Gain=m1
  Gain7 : Gain  Gain=m2
  Gain8 : Gain  Gain=m2*g*l2
  Product{1..3,7..9} (6 alike) : Product
  Product4 : Product  Inputs=4
  Product5 : Product  Inputs=3
  Product6 : Product  Inputs=3
  Sin : Trigonometry
  Sin1 : Trigonometry
  Sin2 : Trigonometry
  Square1 : Math  Operator=square
  T1 : Outport
  wires:
  Constant/1 -> Gain1/1
  Constant2/1 -> Gain2/1
  Cos/1 -> Product2/2
  Gain2/1 -> Product2/1, Product5/1
  Gain1/1 -> Add1/1
  Product2/1 -> Add1/2
  theta2ddot/1 -> Product3/1
  Add1/1 -> Product3/2
  theta1dot/1 -> Product4/3
  theta2dot/1 -> Product4/4, Square1/1
  Sin/1 -> Product4/2, Product5/2
  Gain4/1 -> Product4/1
  Constant3/1 -> Gain4/1
  Square1/1 -> Product5/3
  Constant4/1 -> Gain6/1
  Constant5/1 -> Gain7/1
  Gain7/1 -> Add3/2
  Gain6/1 -> Add3/1
  theta1/1 -> Add4/2, Sin1/1
  Add3/1 -> Product6/1
  Sin1/1 -> Product6/2
  Constant6/1 -> Product6/3
  Constant7/1 -> Gain8/1
  Add4/1 -> Sin2/1
  Gain8/1 -> Product7/1
  Sin2/1 -> Product7/2
  Product3/1 -> Add5/1
  Product4/1 -> Add5/2
  Product5/1 -> Add5/3
  Product6/1 -> Add5/4
  Product7/1 -> Add5/5
  theta2/1 -> Cos1/1, Add4/1, Sin/1, Cos/1
  Constant12/1 -> Product8/2  "X_dd"
  Cos1/1 -> Product8/1
  Constant9/1 -> Add6/3
  Constant10/1 -> Add6/4
  Constant11/1 -> Add6/2
  Product8/1 -> Add6/1
  Add6/1 -> Product1/2
  theta1ddot/1 -> Add2/1
  Product1/1 -> Add5/6
  Add5/1 -> T1/1
  [edotFR1] -> Product9/2
  [lamdaFR1] -> Product9/1
  Product9/1 -> Add2/2
  Add2/1 -> Product1/1

== system singlcontact_control_smc_lqr_mydimes_reaction/Walking Robot/smc+neuro1+reaction/SMC Controllers FR/Equivalent control/SMC equivalent T2 ==
  theta1ddot : Inport
  theta2 : Inport  Port=2
  theta1 : Inport  Port=3
  theta2ddot : Inport  Port=4
  theta1dot : Inport  Port=5
  Add1 : Sum
  Add2 : Sum
  Add4 : Sum
  Add5 : Sum  Inputs=++++
  Constant : Constant  Value=0.5
  Constant1 : Constant  Value=0.3
  Constant2 : Constant  Value=0.5
  Constant3 : Constant
  Gain10 : Gain  Gain=m2*l2^2
  Gain11 : Gain  Gain=m2*l2
  Gain12 : Gain  Gain=g
  Gain13 : Gain  Gain=(1/3)*(m2*(l2^2))
  Gain5 : Gain  Gain=m2*l1*l2
  Product{1..4,7} (5 alike) : Product
  Product6 : Product  Inputs=3
  Sin : Trigonometry
  Square3 : Math  Operator=square
  Trigonometric Function3 : Trigonometry  Operator=cos
  Trigonometric Function4 : Trigonometry
  T2 : Outport
  wires:
  theta2/1 -> Trigonometric Function3/1, Add4/2, Trigonometric Function4/1
  Trigonometric Function3/1 -> Product3/1
  Gain5/1 -> Product3/2, Product6/1
  Product3/1 -> Add2/1
  Gain10/1 -> Add2/2
  Add2/1 -> Product4/2
  theta1ddot/1 -> Product4/1
  Constant/1 -> Gain5/1
  Constant1/1 -> Gain10/1
  Trigonometric Function4/1 -> Product6/2
  theta1dot/1 -> Square3/1
  Square3/1 -> Product6/3
  Constant2/1 -> Gain11/1
  Gain11/1 -> Gain12/1
  Gain12/1 -> Product7/1
  theta1/1 -> Add4/1
  Sin/1 -> Product7/2
  Add4/1 -> Sin/1
  Product4/1 -> Add5/1
  Product6/1 -> Add5/2
  Product7/1 -> Add5/3
  Add5/1 -> T2/1
  Product1/1 -> Add1/1
  [lamdaFR2] -> Product1/2
  [edotFR2] -> Product1/1
  theta2ddot/1 -> Add1/2
  Constant3/1 -> Gain13/1
  Add1/1 -> Product2/2
  Gain13/1 -> Product2/1
  Product2/1 -> Add5/4

== system singlcontact_control_smc_lqr_mydimes_reaction/Walking Robot/smc+neuro1+reaction/SMC Controllers FR/Subsystem2/length from ground ==
  In1 : Inport
  In2 : Inport  Port=2
  Gain1 : Gain  Gain=l1
  Gain3 : Gain  Gain=l1
  Gain4 : Gain  Gain=l2
  Sin : Trigonometry
  Sin1 : Trigonometry
  Sin3 : Trigonometry
  Sum : Sum  Inputs=|++
  Sum2 : Sum  Inputs=|++
  Output : Outport
  Outport : Outport  Port=2
  wires:
  In1/1 -> Sin/1, Sum2/1, Sin1/1
  Sin/1 -> Gain1/1
  Sum/1 -> Outport/1
  Gain4/1 -> Sum/2
  Gain3/1 -> Sum/1
  Sum2/1 -> Sin3/1
  Sin1/1 -> Gain3/1
  Gain1/1 -> Output/1
  Sin3/1 -> Gain4/1
  In2/1 -> Sum2/2

== system singlcontact_control_smc_lqr_mydimes_reaction/Walking Robot/smc+neuro1+reaction/SMC Controllers FR1/Equivalent control/SMC equivalent T1 ==
  theta2 : Inport
  theta1 : Inport  Port=2
  theta2ddot : Inport  Port=3
  theta1dot : Inport  Port=4
  theta2dot : Inport  Port=5
  theta1ddot : Inport  Port=6
  Add{1..4} (4 alike) : Sum
  Add5 : Sum  Inputs=+--+++
  Add6 : Sum  Inputs=++++
  Constant : Constant  Value=0.3
  Constant10 : Constant  Value=m2*l1^2
  Constant11 : Constant  Value=0.3*m1*l1^2
  Constant12 : Constant  Value=m2*l1*l2
  Constant2 : Constant  Value=0.5
  Constant3 : Constant
  Constant4 : Constant  Value=0.5
  Constant5 : Constant
  Constant6 : Constant  Value=g*l1
  Constant7 : Constant  Value=0.5
  Constant9 : Constant  Value=0.3*m2*l2^2
  Cos : Trigonometry  Operator=cos
  Cos1 : Trigonometry  Operator=cos
  Gain1 : Gain  Gain=m2*l2^2
  Gain2 : Gain  Gain=m2*l2*l1
  Gain4 : Gain  Gain=m2*l2*l1
  Gain6 : Gain  Gain=m1
  Gain7 : Gain  Gain=m2
  Gain8 : Gain  Gain=m2*g*l2
  Product{1..3,7..9} (6 alike) : Product
  Product4 : Product  Inputs=4
  Product5 : Product  Inputs=3
  Product6 : Product  Inputs=3
  Sin : Trigonometry
  Sin1 : Trigonometry
  Sin2 : Trigonometry
  Square1 : Math  Operator=square
  T1 : Outport
  wires:
  Add2/1 -> Product1/1
  Product9/1 -> Add2/2
  [lamdaFL1] -> Product9/1
  [edotFL1] -> Product9/2
  Add5/1 -> T1/1
  Product1/1 -> Add5/6
  theta1ddot/1 -> Add2/1
  Add6/1 -> Product1/2
  Product8/1 -> Add6/1
  Constant11/1 -> Add6/2
  Constant10/1 -> Add6/4
  Constant9/1 -> Add6/3
  Cos1/1 -> Product8/1
  Constant12/1 -> Product8/2  "X_dd"
  theta2/1 -> Cos/1, Sin/1, Add4/1, Cos1/1
  Product7/1 -> Add5/5
  Product6/1 -> Add5/4
  Product5/1 -> Add5/3
  Product4/1 -> Add5/2
  Product3/1 -> Add5/1
  Sin2/1 -> Product7/2
  Gain8/1 -> Product7/1
  Add4/1 -> Sin2/1
  Constant7/1 -> Gain8/1
  Constant6/1 -> Product6/3
  Sin1/1 -> Product6/2
  Add3/1 -> Product6/1
  theta1/1 -> Sin1/1, Add4/2
  Gain6/1 -> Add3/1
  Gain7/1 -> Add3/2
  Constant5/1 -> Gain7/1
  Constant4/1 -> Gain6/1
  Square1/1 -> Product5/3
  Constant3/1 -> Gain4/1
  Gain4/1 -> Product4/1
  Sin/1 -> Product5/2, Product4/2
  theta2dot/1 -> Square1/1, Product4/4
  theta1dot/1 -> Product4/3
  Add1/1 -> Product3/2
  theta2ddot/1 -> Product3/1
  Product2/1 -> Add1/2
  Gain1/1 -> Add1/1
  Gain2/1 -> Product5/1, Product2/1
  Cos/1 -> Product2/2
  Constant2/1 -> Gain2/1
  Constant/1 -> Gain1/1

== system singlcontact_control_smc_lqr_mydimes_reaction/Walking Robot/smc+neuro1+reaction/SMC Controllers FR1/Equivalent control/SMC equivalent T2 ==
  theta1ddot : Inport
  theta2 : Inport  Port=2
  theta1 : Inport  Port=3
  theta2ddot : Inport  Port=4
  theta1dot : Inport  Port=5
  Add1 : Sum
  Add2 : Sum
  Add4 : Sum
  Add5 : Sum  Inputs=++++
  Constant : Constant  Value=0.5
  Constant1 : Constant  Value=0.3
  Constant2 : Constant  Value=0.5
  Constant3 : Constant
  Gain10 : Gain  Gain=m2*l2^2
  Gain11 : Gain  Gain=m2*l2
  Gain12 : Gain  Gain=g
  Gain13 : Gain  Gain=(1/3)*(m2*(l2^2))
  Gain5 : Gain  Gain=m2*l1*l2
  Product{1..4,7} (5 alike) : Product
  Product6 : Product  Inputs=3
  Sin : Trigonometry
  Square3 : Math  Operator=square
  Trigonometric Function3 : Trigonometry  Operator=cos
  Trigonometric Function4 : Trigonometry
  T2 : Outport
  wires:
  Product2/1 -> Add5/4
  Gain13/1 -> Product2/1
  Add1/1 -> Product2/2
  Constant3/1 -> Gain13/1
  theta2ddot/1 -> Add1/2
  [edotFL2] -> Product1/1
  [lamdaFL2] -> Product1/2
  Product1/1 -> Add1/1
  Add5/1 -> T2/1
  Product7/1 -> Add5/3
  Product6/1 -> Add5/2
  Product4/1 -> Add5/1
  Add4/1 -> Sin/1
  Sin/1 -> Product7/2
  theta1/1 -> Add4/1
  Gain12/1 -> Product7/1
  Gain11/1 -> Gain12/1
  Constant2/1 -> Gain11/1
  Square3/1 -> Product6/3
  theta1dot/1 -> Square3/1
  Trigonometric Function4/1 -> Product6/2
  Constant1/1 -> Gain10/1
  Constant/1 -> Gain5/1
  theta1ddot/1 -> Product4/1
  Add2/1 -> Product4/2
  Gain10/1 -> Add2/2
  Product3/1 -> Add2/1
  Gain5/1 -> Product6/1, Product3/2
  Trigonometric Function3/1 -> Product3/1
  theta2/1 -> Trigonometric Function4/1, Add4/2, Trigonometric Function3/1

== system singlcontact_control_smc_lqr_mydimes_reaction/Walking Robot/smc+neuro1+reaction/SMC Controllers FR2/Equivalent control/SMC equivalent T1 ==
  theta2 : Inport
  theta1 : Inport  Port=2
  theta2ddot : Inport  Port=3
  theta1dot : Inport  Port=4
  theta2dot : Inport  Port=5
  theta1ddot : Inport  Port=6
  Add{1..4} (4 alike) : Sum
  Add5 : Sum  Inputs=+--+++
  Add6 : Sum  Inputs=++++
  Constant : Constant  Value=0.3
  Constant10 : Constant  Value=m2*l1^2
  Constant11 : Constant  Value=0.3*m1*l1^2
  Constant12 : Constant  Value=m2*l1*l2
  Constant2 : Constant  Value=0.5
  Constant3 : Constant
  Constant4 : Constant  Value=0.5
  Constant5 : Constant
  Constant6 : Constant  Value=g*l1
  Constant7 : Constant  Value=0.5
  Constant9 : Constant  Value=0.3*m2*l2^2
  Cos : Trigonometry  Operator=cos
  Cos1 : Trigonometry  Operator=cos
  Gain1 : Gain  Gain=m2*l2^2
  Gain2 : Gain  Gain=m2*l2*l1
  Gain4 : Gain  Gain=m2*l2*l1
  Gain6 : Gain  Gain=m1
  Gain7 : Gain  Gain=m2
  Gain8 : Gain  Gain=m2*g*l2
  Product{1..3,7..9} (6 alike) : Product
  Product4 : Product  Inputs=4
  Product5 : Product  Inputs=3
  Product6 : Product  Inputs=3
  Sin : Trigonometry
  Sin1 : Trigonometry
  Sin2 : Trigonometry
  Square1 : Math  Operator=square
  T1 : Outport
  wires:
  Constant/1 -> Gain1/1
  Constant2/1 -> Gain2/1
  Cos/1 -> Product2/2
  Gain2/1 -> Product2/1, Product5/1
  Gain1/1 -> Add1/1
  Product2/1 -> Add1/2
  theta2ddot/1 -> Product3/1
  Add1/1 -> Product3/2
  theta1dot/1 -> Product4/3
  theta2dot/1 -> Product4/4, Square1/1
  Sin/1 -> Product4/2, Product5/2
  Gain4/1 -> Product4/1
  Constant3/1 -> Gain4/1
  Square1/1 -> Product5/3
  Constant4/1 -> Gain6/1
  Constant5/1 -> Gain7/1
  Gain7/1 -> Add3/2
  Gain6/1 -> Add3/1
  theta1/1 -> Add4/2, Sin1/1
  Add3/1 -> Product6/1
  Sin1/1 -> Product6/2
  Constant6/1 -> Product6/3
  Constant7/1 -> Gain8/1
  Add4/1 -> Sin2/1
  Gain8/1 -> Product7/1
  Sin2/1 -> Product7/2
  Product3/1 -> Add5/1
  Product4/1 -> Add5/2
  Product5/1 -> Add5/3
  Product6/1 -> Add5/4
  Product7/1 -> Add5/5
  theta2/1 -> Cos1/1, Add4/1, Sin/1, Cos/1
  Constant12/1 -> Product8/2  "X_dd"
  Cos1/1 -> Product8/1
  Constant9/1 -> Add6/3
  Constant10/1 -> Add6/4
  Constant11/1 -> Add6/2
  Product8/1 -> Add6/1
  Add6/1 -> Product1/2
  theta1ddot/1 -> Add2/1
  Product1/1 -> Add5/6
  Add5/1 -> T1/1
  [edotBR1] -> Product9/2
  [lamdaBR1] -> Product9/1
  Product9/1 -> Add2/2
  Add2/1 -> Product1/1

== system singlcontact_control_smc_lqr_mydimes_reaction/Walking Robot/smc+neuro1+reaction/SMC Controllers FR2/Equivalent control/SMC equivalent T2 ==
  theta1ddot : Inport
  theta2 : Inport  Port=2
  theta1 : Inport  Port=3
  theta2ddot : Inport  Port=4
  theta1dot : Inport  Port=5
  Add1 : Sum
  Add2 : Sum
  Add4 : Sum
  Add5 : Sum  Inputs=++++
  Constant : Constant  Value=0.5
  Constant1 : Constant  Value=0.3
  Constant2 : Constant  Value=0.5
  Constant3 : Constant
  Gain10 : Gain  Gain=m2*l2^2
  Gain11 : Gain  Gain=m2*l2
  Gain12 : Gain  Gain=g
  Gain13 : Gain  Gain=(1/3)*(m2*(l2^2))
  Gain5 : Gain  Gain=m2*l1*l2
  Product{1..4,7} (5 alike) : Product
  Product6 : Product  Inputs=3
  Sin : Trigonometry
  Square3 : Math  Operator=square
  Trigonometric Function3 : Trigonometry  Operator=cos
  Trigonometric Function4 : Trigonometry
  T2 : Outport
  wires:
  theta2/1 -> Trigonometric Function3/1, Add4/2, Trigonometric Function4/1
  Trigonometric Function3/1 -> Product3/1
  Gain5/1 -> Product3/2, Product6/1
  Product3/1 -> Add2/1
  Gain10/1 -> Add2/2
  Add2/1 -> Product4/2
  theta1ddot/1 -> Product4/1
  Constant/1 -> Gain5/1
  Constant1/1 -> Gain10/1
  Trigonometric Function4/1 -> Product6/2
  theta1dot/1 -> Square3/1
  Square3/1 -> Product6/3
  Constant2/1 -> Gain11/1
  Gain11/1 -> Gain12/1
  Gain12/1 -> Product7/1
  theta1/1 -> Add4/1
  Sin/1 -> Product7/2
  Add4/1 -> Sin/1
  Product4/1 -> Add5/1
  Product6/1 -> Add5/2
  Product7/1 -> Add5/3
  Add5/1 -> T2/1
  Product1/1 -> Add1/1
  [lamdaBR2] -> Product1/2
  [edotBR2] -> Product1/1
  theta2ddot/1 -> Add1/2
  Constant3/1 -> Gain13/1
  Add1/1 -> Product2/2
  Gain13/1 -> Product2/1
  Product2/1 -> Add5/4

== system singlcontact_control_smc_lqr_mydimes_reaction/Walking Robot/smc+neuro1+reaction/SMC Controllers FR3/Equivalent control/SMC equivalent T1 ==
  theta2 : Inport
  theta1 : Inport  Port=2
  theta2ddot : Inport  Port=3
  theta1dot : Inport  Port=4
  theta2dot : Inport  Port=5
  theta1ddot : Inport  Port=6
  Add{1..4} (4 alike) : Sum
  Add5 : Sum  Inputs=+--+++
  Add6 : Sum  Inputs=++++
  Constant : Constant  Value=0.3
  Constant10 : Constant  Value=m2*l1^2
  Constant11 : Constant  Value=0.3*m1*l1^2
  Constant12 : Constant  Value=m2*l1*l2
  Constant2 : Constant  Value=0.5
  Constant3 : Constant
  Constant4 : Constant  Value=0.5
  Constant5 : Constant
  Constant6 : Constant  Value=g*l1
  Constant7 : Constant  Value=0.5
  Constant9 : Constant  Value=0.3*m2*l2^2
  Cos : Trigonometry  Operator=cos
  Cos1 : Trigonometry  Operator=cos
  Gain1 : Gain  Gain=m2*l2^2
  Gain2 : Gain  Gain=m2*l2*l1
  Gain4 : Gain  Gain=m2*l2*l1
  Gain6 : Gain  Gain=m1
  Gain7 : Gain  Gain=m2
  Gain8 : Gain  Gain=m2*g*l2
  Product{1..3,7..9} (6 alike) : Product
  Product4 : Product  Inputs=4
  Product5 : Product  Inputs=3
  Product6 : Product  Inputs=3
  Sin : Trigonometry
  Sin1 : Trigonometry
  Sin2 : Trigonometry
  Square1 : Math  Operator=square
  T1 : Outport
  wires:
  Add2/1 -> Product1/1
  Product9/1 -> Add2/2
  [lamdaBL1] -> Product9/1
  [edotBL1] -> Product9/2
  Add5/1 -> T1/1
  Product1/1 -> Add5/6
  theta1ddot/1 -> Add2/1
  Add6/1 -> Product1/2
  Product8/1 -> Add6/1
  Constant11/1 -> Add6/2
  Constant10/1 -> Add6/4
  Constant9/1 -> Add6/3
  Cos1/1 -> Product8/1
  Constant12/1 -> Product8/2  "X_dd"
  theta2/1 -> Cos/1, Sin/1, Add4/1, Cos1/1
  Product7/1 -> Add5/5
  Product6/1 -> Add5/4
  Product5/1 -> Add5/3
  Product4/1 -> Add5/2
  Product3/1 -> Add5/1
  Sin2/1 -> Product7/2
  Gain8/1 -> Product7/1
  Add4/1 -> Sin2/1
  Constant7/1 -> Gain8/1
  Constant6/1 -> Product6/3
  Sin1/1 -> Product6/2
  Add3/1 -> Product6/1
  theta1/1 -> Sin1/1, Add4/2
  Gain6/1 -> Add3/1
  Gain7/1 -> Add3/2
  Constant5/1 -> Gain7/1
  Constant4/1 -> Gain6/1
  Square1/1 -> Product5/3
  Constant3/1 -> Gain4/1
  Gain4/1 -> Product4/1
  Sin/1 -> Product5/2, Product4/2
  theta2dot/1 -> Square1/1, Product4/4
  theta1dot/1 -> Product4/3
  Add1/1 -> Product3/2
  theta2ddot/1 -> Product3/1
  Product2/1 -> Add1/2
  Gain1/1 -> Add1/1
  Gain2/1 -> Product5/1, Product2/1
  Cos/1 -> Product2/2
  Constant2/1 -> Gain2/1
  Constant/1 -> Gain1/1

== system singlcontact_control_smc_lqr_mydimes_reaction/Walking Robot/smc+neuro1+reaction/SMC Controllers FR3/Equivalent control/SMC equivalent T2 ==
  theta1ddot : Inport
  theta2 : Inport  Port=2
  theta1 : Inport  Port=3
  theta2ddot : Inport  Port=4
  theta1dot : Inport  Port=5
  Add1 : Sum
  Add2 : Sum
  Add4 : Sum
  Add5 : Sum  Inputs=++++
  Constant : Constant  Value=0.5
  Constant1 : Constant  Value=0.3
  Constant2 : Constant  Value=0.5
  Constant3 : Constant
  Gain10 : Gain  Gain=m2*l2^2
  Gain11 : Gain  Gain=m2*l2
  Gain12 : Gain  Gain=g
  Gain13 : Gain  Gain=(1/3)*(m2*(l2^2))
  Gain5 : Gain  Gain=m2*l1*l2
  Product{1..4,7} (5 alike) : Product
  Product6 : Product  Inputs=3
  Sin : Trigonometry
  Square3 : Math  Operator=square
  Trigonometric Function3 : Trigonometry  Operator=cos
  Trigonometric Function4 : Trigonometry
  T2 : Outport
  wires:
  Product2/1 -> Add5/4
  Gain13/1 -> Product2/1
  Add1/1 -> Product2/2
  Constant3/1 -> Gain13/1
  theta2ddot/1 -> Add1/2
  [edotBL2] -> Product1/1
  [lamdaBL2] -> Product1/2
  Product1/1 -> Add1/1
  Add5/1 -> T2/1
  Product7/1 -> Add5/3
  Product6/1 -> Add5/2
  Product4/1 -> Add5/1
  Add4/1 -> Sin/1
  Sin/1 -> Product7/2
  theta1/1 -> Add4/1
  Gain12/1 -> Product7/1
  Gain11/1 -> Gain12/1
  Constant2/1 -> Gain11/1
  Square3/1 -> Product6/3
  theta1dot/1 -> Square3/1
  Trigonometric Function4/1 -> Product6/2
  Constant1/1 -> Gain10/1
  Constant/1 -> Gain5/1
  theta1ddot/1 -> Product4/1
  Add2/1 -> Product4/2
  Gain10/1 -> Add2/2
  Product3/1 -> Add2/1
  Gain5/1 -> Product6/1, Product3/2
  Trigonometric Function3/1 -> Product3/1
  theta2/1 -> Trigonometric Function4/1, Add4/2, Trigonometric Function3/1
